simulink model "MODEL_nieliniowy_prevprevprev"  (R2020b)
settings: Solver=VariableStepAuto  StartTime=0.0  StopTime=1200  RelTol=1e-3
values from neighbouring files (symbols this model uses):
  c1 = 1    [zadanie_inaczej.m]
  c2 = 2    [zadanie_inaczej.m]
  K = 0.02    [zadanie_inaczej.m]
  S = 1    [zadanie_inaczej.m]
settings Model: PauseTimes=0  Creator=Adam  LastModifiedBy=Adam

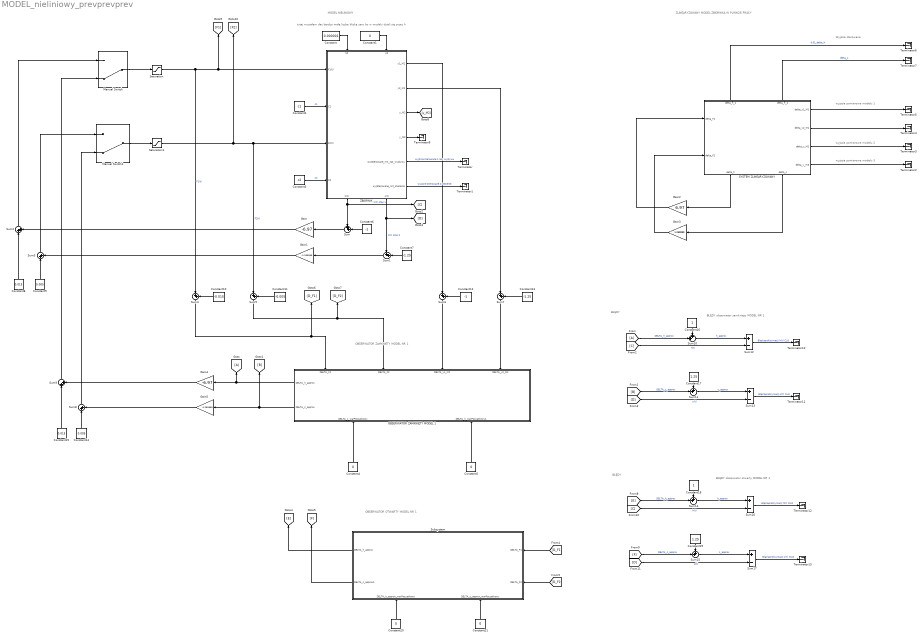
== system MODEL_nieliniowy_prevprevprev ==
  note: BŁĘDY obserwator zamknięty MODEL NR 1
  note: OBSERWATOR ZAMKNIETY MODEL NR 1
  note: BŁĘDY
  note: tutaj musiałem dać bardzo małą liczbe bliską zero bo w modelu dzieli się przez h
  note: wyjscia pomiarowe modelu 3
  note: ZLINEARYZOWANY MODEL ZBIORNIKA W PUNKCIE PRACY
  note: wyjscia pomiarowe modelu 1
  note: wyjscia pomiarowe modelu 2
  note: Wyjścia sterowane
  note: MODEL NIELINIOWY
  note: BŁĘDY
  note: BŁĘDY obserwator otwarty
      | MODEL NR 1
  note: OBSERWATOR OTWARTY MODEL NR 1
  Constant : Constant  Value=0.000001
  Constant{1,4..5,20..21} (5 alike) : Constant  Value=0
  Constant10 : Constant  Value=-0.015
  Constant11 : Constant  Value=-0.005
  Constant12 : Constant  Value=-1
  Constant13 : Constant  Value=-1.25
  Constant14 : Constant  Value=0.005
  Constant15 : Constant  Value=0.015
  Constant16 : Constant
  Constant17 : Constant  Value=1.25
  Constant18 : Constant
  Constant19 : Constant  Value=1.25
  Constant2 : Constant  Value=c1
  Constant3 : Constant  Value=c2
  Constant6 : Constant  Value=-1
  Constant7 : Constant  Value=-1.25
  Constant8 : Constant  Value=0.015
  Constant9 : Constant  Value=0.005
  Gain : Gain  Gain=-6.97
  Gain1 : Gain  Gain=-1.269999
  Gain2 : Gain  Gain=6.97
  Gain3 : Gain  Gain=1.269999
  Gain4 : Gain  Gain=-6.97
  Gain5 : Gain  Gain=-1.269999
  Manual Switch : ManualSwitch  CurrentSetting=0
  Manual Switch1 : ManualSwitch  CurrentSetting=0
  OBSERWATOR ZAMKNIĘTY MODEL 1 : Subsystem
      settings: PortSchema="{\"entries\":[{\"content\":{\"sides\":[{\"content\":{\"connectorIds\":[]},\"type\":\"ConnectorPlacement.EquallySpacedRectSide\",\"uuid\":\"df9a0dc1-4b9c-40dc-a757-6b1a6b9aa6ed\"},{\"content\":{\"connectorIds\":[\"Out1\",\"Out2\"],\"side\":\"RIGHT\"},\"type\":\"ConnectorPlacement.EquallySpacedRectSide\",\"uuid\":\"5cba16cf-a15e-4045-92be-3e6ecad2ae7f\"},{\"content\":{\"connectorIds\":[\"In1\",\"In2\",\"In3\",\"In4\"],\"side\":\"TOP\"},\"type\":\"ConnectorPlacement.EquallySpacedRectSide\",\"uuid\":\"e348609f-8070-4092-8204-65a83adf26dd\"},{\"content\":{\"connectorIds\":[\"In5\",\"In6\"],\"side\":\"BOTTOM\"},\"type\":\"ConnectorPlacement.EquallySpacedRectSide\",\"uuid\":\"61fc9fd5-86f3-4303-bf38-07e595d55bb3\"},{\"content\":{\"connectorIds\":[],\"side\":\"HIDDEN\"},\"type\":\"ConnectorPlacement.EquallySpacedRectSide\",\"uuid\":\"65a64511-4a73-4e57-a778-b63fa28d7d79\"}]},\"type\":\"ConnectorPlacement.EquallySpacedConnector\",\"uuid\":\"74f27241-a0e0-45b7-b881-233bfa2226d6\"}],\"packageUris\":[\"http://schema.mathworks.com/mf0/Connector/R2020b\"],\"version\":\"1.0\"}"
  SYSTEM ZLINEARYZOWANY : Subsystem
      settings: PortSchema="{\"entries\":[{\"content\":{\"sides\":[{\"content\":{\"connectorIds\":[\"In1\",\"In2\"]},\"type\":\"ConnectorPlacement.EquallySpacedRectSide\",\"uuid\":\"d54e25d2-cd73-45e0-9808-ca3ea5dc6cf7\"},{\"content\":{\"connectorIds\":[\"Out1\",\"Out2\",\"Out3\",\"Out4\"],\"side\":\"RIGHT\"},\"type\":\"ConnectorPlacement.EquallySpacedRectSide\",\"uuid\":\"8f74ab67-fea9-4695-8f57-14f1d1e6aeae\"},{\"content\":{\"connectorIds\":[\"Out7\",\"Out8\"],\"side\":\"TOP\"},\"type\":\"ConnectorPlacement.EquallySpacedRectSide\",\"uuid\":\"7e2d5216-70d7-4fc4-9048-f9922785c559\"},{\"content\":{\"connectorIds\":[\"Out5\",\"Out6\"],\"side\":\"BOTTOM\"},\"type\":\"ConnectorPlacement.EquallySpacedRectSide\",\"uuid\":\"2e3112e0-8f75-4fde-8abe-6ce63d8f82f0\"},{\"content\":{\"connectorIds\":[],\"side\":\"HIDDEN\"},\"type\":\"ConnectorPlacement.EquallySpacedRectSide\",\"uuid\":\"0c231cea-7ad8-44fc-a940-5c2cadec50e3\"}]},\"type\":\"ConnectorPlacement.EquallySpacedConnector\",\"uuid\":\"51c5d8a6-0e0c-4ace-bfb7-5845e71f886b\"}],\"packageUris\":[\"http://schema.mathworks.com/mf0/Connector/R2020b\"],\"version\":\"1.0\"}"
  Saturation : Saturate  UpperLimit=inf  LowerLimit=0
  Saturation1 : Saturate  UpperLimit=inf  LowerLimit=0
  Subsystem : Subsystem
      settings: PortSchema="{\"entries\":[{\"content\":{\"sides\":[{\"content\":{\"connectorIds\":[\"In1\",\"In2\"]},\"type\":\"ConnectorPlacement.EquallySpacedRectSide\",\"uuid\":\"9da57aff-d8ed-41ac-be0f-7bb7d22a2d6d\"},{\"content\":{\"connectorIds\":[\"Out1\",\"Out2\"],\"side\":\"RIGHT\"},\"type\":\"ConnectorPlacement.EquallySpacedRectSide\",\"uuid\":\"4a485f9a-c196-4acf-9f6f-00c6dbb16d48\"},{\"content\":{\"connectorIds\":[],\"side\":\"TOP\"},\"type\":\"ConnectorPlacement.EquallySpacedRectSide\",\"uuid\":\"007a8443-3490-401f-88cc-683f6a14c27c\"},{\"content\":{\"connectorIds\":[\"In3\",\"In4\"],\"side\":\"BOTTOM\"},\"type\":\"ConnectorPlacement.EquallySpacedRectSide\",\"uuid\":\"09129c57-b904-461c-b339-9340df3751d4\"},{\"content\":{\"connectorIds\":[],\"side\":\"HIDDEN\"},\"type\":\"ConnectorPlacement.EquallySpacedRectSide\",\"uuid\":\"f4f5cd58-23cc-4937-8552-2264c9543629\"}]},\"type\":\"ConnectorPlacement.EquallySpacedConnector\",\"uuid\":\"c4e5adba-5bf6-49ba-a33f-504984928f5e\"}],\"packageUris\":[\"http://schema.mathworks.com/mf0/Connector/R2020b\"],\"version\":\"1.0\"}"
  Sum{,1,10..11,14..15} (6 alike) : Sum  Inputs=++|
  Sum{12..13,16..17} (4 alike) : Sum  Inputs=+-
  Sum{2..9} (8 alike) : Sum  Inputs=|++
  Terminator{,1..7,9..13} (13 alike) : Terminator
  ZBIORNIK : Subsystem
      settings: PortSchema="{\"entries\":[{\"content\":{\"sides\":[{\"content\":{\"connectorIds\":[\"In1\",\"In2\",\"In3\",\"In4\"]},\"type\":\"ConnectorPlacement.EquallySpacedRectSide\",\"uuid\":\"d7534cdc-3a83-4663-9669-478cefb7ba54\"},{\"content\":{\"connectorIds\":[\"Out1\",\"Out2\",\"Out3\",\"Out4\",\"Out5\",\"Out6\"],\"side\":\"RIGHT\"},\"type\":\"ConnectorPlacement.EquallySpacedRectSide\",\"uuid\":\"43aa4112-be2a-4a64-a360-86159253405e\"},{\"content\":{\"connectorIds\":[\"In5\",\"In6\"],\"side\":\"TOP\"},\"type\":\"ConnectorPlacement.EquallySpacedRectSide\",\"uuid\":\"a87f647c-d073-49ff-8fa7-c7401791c269\"},{\"content\":{\"connectorIds\":[\"Out7\",\"Out8\"],\"side\":\"BOTTOM\"},\"type\":\"ConnectorPlacement.EquallySpacedRectSide\",\"uuid\":\"6d6aa66b-079d-45b1-a0b1-1cea6131b53f\"},{\"content\":{\"connectorIds\":[],\"side\":\"HIDDEN\"},\"type\":\"ConnectorPlacement.EquallySpacedRectSide\",\"uuid\":\"1d6cc66c-e8b9-4690-8052-ee4d3cbcc1b2\"}]},\"type\":\"ConnectorPlacement.EquallySpacedConnector\",\"uuid\":\"a7312018-d894-48d8-963b-edf04426afa5\"}],\"packageUris\":[\"http://schema.mathworks.com/mf0/Connector/R2020b\"],\"version\":\"1.0\"}"
  wires:
  Constant2/1 -> ZBIORNIK/2(C1)  "c1"
  Constant3/1 -> ZBIORNIK/4(C2)  "c2"
  Constant1/1 -> ZBIORNIK/6(c0)
  Constant/1 -> ZBIORNIK/5(h0)
  SYSTEM ZLINEARYZOWANY/7(delta_fi_1) -> Terminator6/1  "0.01_delta_h"
  SYSTEM ZLINEARYZOWANY/1(delta_y1_M1) -> Terminator5/1
  SYSTEM ZLINEARYZOWANY/2(delta_y2_M1) -> Terminator4/1
  SYSTEM ZLINEARYZOWANY/3(delta_y_M2) -> Terminator3/1
  SYSTEM ZLINEARYZOWANY/4(delta_y_m3) -> Terminator2/1
  SYSTEM ZLINEARYZOWANY/8(delta_fi_2) -> Terminator7/1  "delta_c"
  ZBIORNIK/7(h(t)) -> [C], Sum/1  "h(t) stan 1"
  Sum/1 -> Gain/1
  Constant6/1 -> Sum/2
  Constant7/1 -> Sum1/2
  ZBIORNIK/8(c(t)) -> Sum1/1, [D]  "c(t) stan 2"
  Sum1/1 -> Gain1/1
  Gain/1 -> Sum2/2
  Gain1/1 -> Sum3/2
  Constant8/1 -> Sum2/1
  Constant9/1 -> Sum3/1
  ZBIORNIK/5(wyjSterowane_nr1_nat_wyplywu) -> Terminator/1  "wyjście sterowane 1 nat. wyplywu"
  ZBIORNIK/6(wyjSterowane_nr2_stezenie) -> Terminator1/1  "wyjście sterowane 2 stezenie"
  SYSTEM ZLINEARYZOWANY/5(delta_h) -> Gain2/1
  SYSTEM ZLINEARYZOWANY/6(delta_c) -> Gain3/1
  Gain2/1 -> SYSTEM ZLINEARYZOWANY/1(delta_F1)
  Gain3/1 -> SYSTEM ZLINEARYZOWANY/2(delta_F2)
  Saturation/1 -> [F1], ZBIORNIK/1(F1(t)), Sum4/1  "F1(t)"
  Manual Switch/1 -> Saturation/1
  Manual Switch1/1 -> Saturation1/1
  Saturation1/1 -> Sum5/1, ZBIORNIK/3(F2(t)), [F2]  "F2(t)"
  Constant10/1 -> Sum4/2
  Constant11/1 -> Sum5/2
  Sum4/1 -> [D_F1], OBSERWATOR ZAMKNIĘTY MODEL 1/4(DELTA_F1)
  Sum5/1 -> OBSERWATOR ZAMKNIĘTY MODEL 1/3(DELTA_F2), [D_F2]
  Constant12/1 -> Sum6/2
  Constant13/1 -> Sum7/2
  ZBIORNIK/1(y1_M1) -> Sum6/1
  ZBIORNIK/2(y2_M1) -> Sum7/1
  Sum6/1 -> OBSERWATOR ZAMKNIĘTY MODEL 1/2(DELTA_y1_M1)
  Sum7/1 -> OBSERWATOR ZAMKNIĘTY MODEL 1/1(DELTA_y2_M2)
  OBSERWATOR ZAMKNIĘTY MODEL 1/2(DELTA_c_approx) -> [B], Gain5/1
  OBSERWATOR ZAMKNIĘTY MODEL 1/1(DELTA_h_approx) -> [A], Gain4/1
  Constant14/1 -> Sum8/1
  Gain5/1 -> Sum8/2
  Constant15/1 -> Sum9/1
  Gain4/1 -> Sum9/2
  Sum2/1 -> Manual Switch/1
  Sum3/1 -> Manual Switch1/1
  Sum9/1 -> Manual Switch/2
  Sum8/1 -> Manual Switch1/2
  Constant4/1 -> OBSERWATOR ZAMKNIĘTY MODEL 1/6(DELTA_c_warPoczatkowy)
  Constant5/1 -> OBSERWATOR ZAMKNIĘTY MODEL 1/5(DELTA_h_warPoczatkowy1)
  ZBIORNIK/3(y_M2) -> [y_M2]
  ZBIORNIK/4(y_M3) -> Terminator9/1
  [A] -> Sum10/2  "DELTA_h_approx"
  [B] -> Sum11/2  "DELTA_c_approx"
  [C] -> Sum12/2  "h(t)"
  [D] -> Sum13/2  "c(t)"
  Constant16/1 -> Sum10/1
  Constant17/1 -> Sum11/1
  Sum10/1 -> Sum12/1  "h_approx"
  Sum11/1 -> Sum13/1  "c_approx"
  Sum13/1 -> Terminator11/1  "Błąd aproksymacji c(t) CLO"
  Sum12/1 -> Terminator10/1  "Błąd aproksymacji h(t) CLO"
  Subsystem/1(DELTA_h_approx) -> [E]
  Subsystem/2(DELTA_c_approx1) -> [F]
  [D_F1] -> Subsystem/1(DELTA_F1)
  [D_F2] -> Subsystem/2(DELTA_F2)
  Sum16/1 -> Terminator12/1  "Błąd aproksymacji h(t) OLO"
  Sum14/1 -> Sum16/1  "h_approx"
  Constant18/1 -> Sum14/1
  Sum15/1 -> Sum17/1  "c_approx"
  Constant19/1 -> Sum15/1
  [D] -> Sum17/2  "c(t)"
  Sum17/1 -> Terminator13/1  "Błąd aproksymacji c(t) OLO"
  [C] -> Sum16/2  "h(t)"
  [E] -> Sum14/2  "DELTA_h_approx"
  [F] -> Sum15/2  "DELTA_c_approx"
  Constant20/1 -> Subsystem/4(DELTA_h_approx_warPoczatkowy)
  Constant21/1 -> Subsystem/3(DELTA_c_approx_warPoczatkowy)

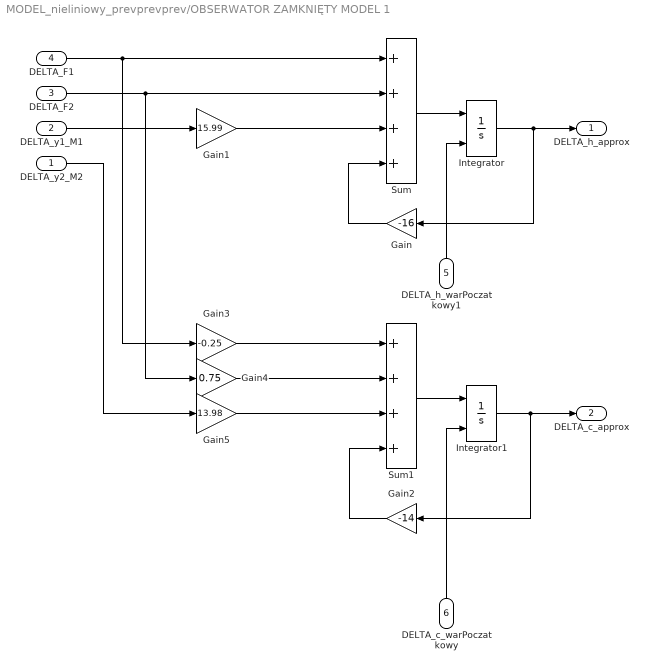
== system MODEL_nieliniowy_prevprevprev/OBSERWATOR ZAMKNIĘTY MODEL 1 ==
  DELTA_y2_M2 : Inport
  DELTA_y1_M1 : Inport  Port=2
  DELTA_F2 : Inport  Port=3
  DELTA_F1 : Inport  Port=4
  DELTA_h_warPoczatkowy1 : Inport  Port=5
  DELTA_c_warPoczatkowy : Inport  Port=6
  Gain : Gain  Gain=-16
  Gain1 : Gain  Gain=15.99
  Gain2 : Gain  Gain=-14
  Gain3 : Gain  Gain=-0.25
  Gain4 : Gain  Gain=0.75
  Gain5 : Gain  Gain=13.98
  Integrator : Integrator  InitialConditionSource=external
  Integrator1 : Integrator  InitialConditionSource=external
  Sum : Sum  Inputs=++++
  Sum1 : Sum  Inputs=++++
  DELTA_h_approx : Outport
  DELTA_c_approx : Outport  Port=2
  wires:
  Integrator/1 -> DELTA_h_approx/1, Gain/1
  Sum/1 -> Integrator/1
  Gain/1 -> Sum/4
  DELTA_F1/1 -> Gain3/1, Sum/1
  DELTA_F2/1 -> Sum/2, Gain4/1
  DELTA_y1_M1/1 -> Gain1/1
  Gain1/1 -> Sum/3
  Integrator1/1 -> DELTA_c_approx/1, Gain2/1
  Sum1/1 -> Integrator1/1
  Gain2/1 -> Sum1/4
  Gain3/1 -> Sum1/1
  Gain4/1 -> Sum1/2
  DELTA_y2_M2/1 -> Gain5/1
  Gain5/1 -> Sum1/3
  DELTA_c_warPoczatkowy/1 -> Integrator1/2
  DELTA_h_warPoczatkowy1/1 -> Integrator/2

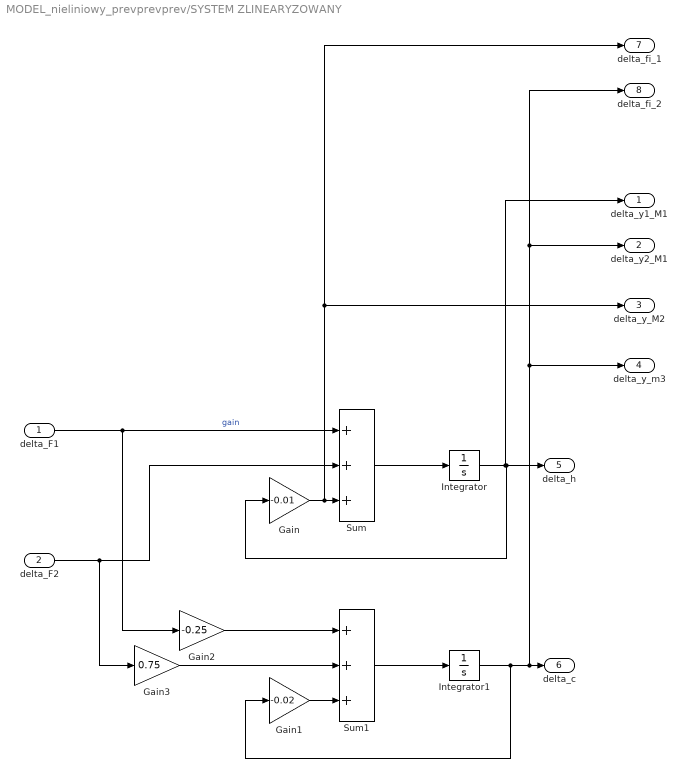
== system MODEL_nieliniowy_prevprevprev/SYSTEM ZLINEARYZOWANY ==
  delta_F1 : Inport
  delta_F2 : Inport  Port=2
  Gain : Gain  Gain=-0.01
  Gain1 : Gain  Gain=-0.02
  Gain2 : Gain  Gain=-0.25
  Gain3 : Gain  Gain=0.75
  Integrator : Integrator
  Integrator1 : Integrator
  Sum : Sum  Inputs=+++
  Sum1 : Sum  Inputs=+++
  delta_y1_M1 : Outport
  delta_y2_M1 : Outport  Port=2
  delta_y_M2 : Outport  Port=3
  delta_y_m3 : Outport  Port=4
  delta_h : Outport  Port=5
  delta_c : Outport  Port=6
  delta_fi_1 : Outport  Port=7
  delta_fi_2 : Outport  Port=8
  wires:
  Integrator1/1 -> delta_y_m3/1, delta_y2_M1/1, delta_fi_2/1, delta_c/1, Gain1/1
  Integrator/1 -> delta_y1_M1/1, Gain/1, delta_h/1
  Gain/1 -> delta_y_M2/1, delta_fi_1/1, Sum/3
  Sum/1 -> Integrator/1
  delta_F1/1 -> Gain2/1, Sum/1  "gain"
  delta_F2/1 -> Gain3/1, Sum/2
  Sum1/1 -> Integrator1/1
  Gain1/1 -> Sum1/3
  Gain2/1 -> Sum1/1
  Gain3/1 -> Sum1/2

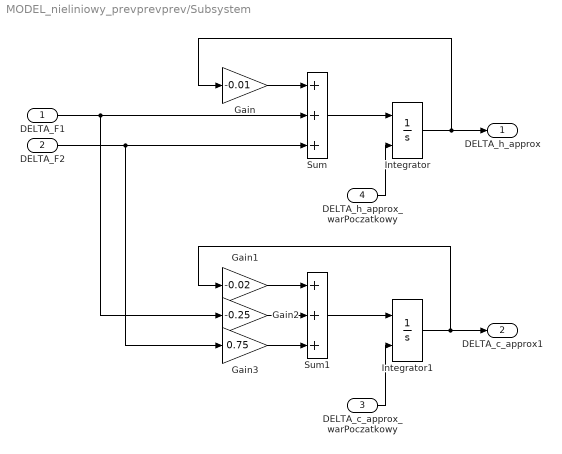
== system MODEL_nieliniowy_prevprevprev/Subsystem ==
  DELTA_F1 : Inport
  DELTA_F2 : Inport  Port=2
  DELTA_c_approx_warPoczatkowy : Inport  Port=3
  DELTA_h_approx_warPoczatkowy : Inport  Port=4
  Gain : Gain  Gain=-0.01
  Gain1 : Gain  Gain=-0.02
  Gain2 : Gain  Gain=-0.25
  Gain3 : Gain  Gain=0.75
  Integrator : Integrator  InitialConditionSource=external
  Integrator1 : Integrator  InitialConditionSource=external
  Sum : Sum  Inputs=+++
  Sum1 : Sum  Inputs=+++
  DELTA_h_approx : Outport
  DELTA_c_approx1 : Outport  Port=2
  wires:
  Gain/1 -> Sum/1
  Sum/1 -> Integrator/1
  Integrator/1 -> Gain/1, DELTA_h_approx/1
  DELTA_F1/1 -> Gain2/1, Sum/2
  DELTA_F2/1 -> Gain3/1, Sum/3
  Sum1/1 -> Integrator1/1
  Integrator1/1 -> Gain1/1, DELTA_c_approx1/1
  Gain1/1 -> Sum1/1
  Gain2/1 -> Sum1/2
  Gain3/1 -> Sum1/3
  DELTA_h_approx_warPoczatkowy/1 -> Integrator/2
  DELTA_c_approx_warPoczatkowy/1 -> Integrator1/2

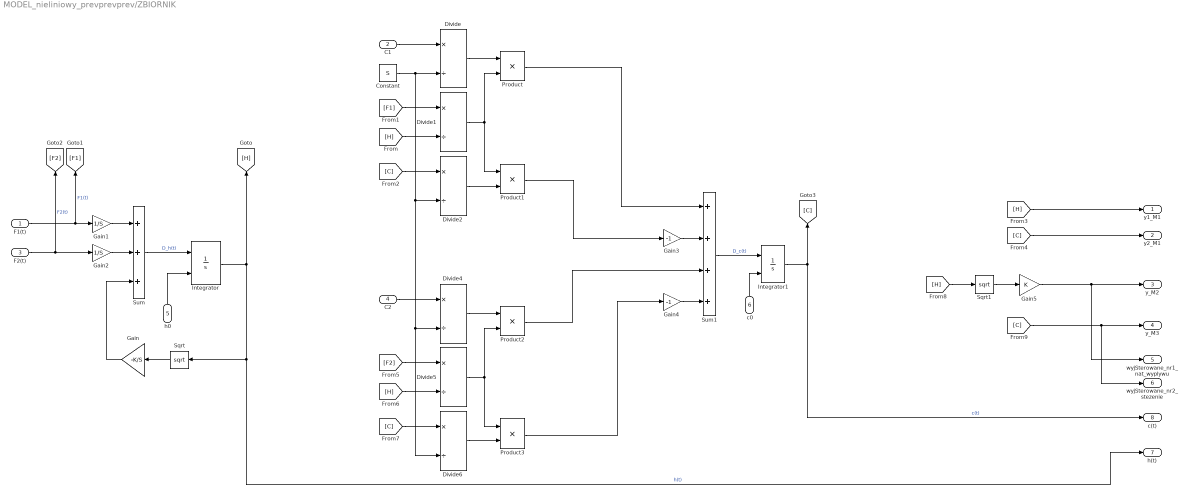
== system MODEL_nieliniowy_prevprevprev/ZBIORNIK ==
  F1(t) : Inport
  C1 : Inport  Port=2
  F2(t) : Inport  Port=3
  C2 : Inport  Port=4
  h0 : Inport  Port=5
  c0 : Inport  Port=6
  Constant : Constant  Value=S
  Divide{,1..2,4..6} (6 alike) : Product  Inputs=*/
  Gain : Gain  Gain=-K/S
  Gain1 : Gain  Gain=1/S
  Gain2 : Gain  Gain=1/S
  Gain3 : Gain  Gain=-1
  Gain4 : Gain  Gain=-1
  Gain5 : Gain  Gain=K
  Integrator : Integrator  InitialConditionSource=external
  Integrator1 : Integrator  InitialConditionSource=external
  Product{,1..3} (4 alike) : Product
  Sqrt : Sqrt  OutputSignalType=real  SaturateOnIntegerOverflow=on
  Sqrt1 : Sqrt  SaturateOnIntegerOverflow=on
  Sum : Sum  Inputs=+++
  Sum1 : Sum  Inputs=++++
  y1_M1 : Outport
  y2_M1 : Outport  Port=2
  y_M2 : Outport  Port=3
  y_M3 : Outport  Port=4
  wyjSterowane_nr1_nat_wyplywu : Outport  Port=5
  wyjSterowane_nr2_stezenie : Outport  Port=6
  h(t) : Outport  Port=7
  c(t) : Outport  Port=8
  wires:
  C2/1 -> Divide4/1
  Product1/1 -> Gain3/1
  Product2/1 -> Sum1/3
  Divide5/1 -> Product3/1, Product2/2
  Gain4/1 -> Sum1/4
  [F2] -> Divide5/1
  Constant/1 -> Divide2/2, Divide4/2, Divide6/2, Divide/2
  C1/1 -> Divide/1
  Sum1/1 -> Integrator1/1  "D_c(t)"
  Product3/1 -> Gain4/1
  F1(t)/1 -> Gain1/1, [F1]  "F1(t)"
  [H] -> Divide1/2
  Gain1/1 -> Sum/1
  F2(t)/1 -> Gain2/1, [F2]  "F2(t)"
  Gain3/1 -> Sum1/2
  [C] -> Divide6/1
  Sum/1 -> Integrator/1  "D_h(t)"
  Divide4/1 -> Product2/1
  Sqrt/1 -> Gain/1
  Integrator1/1 -> [C], c(t)/1  "c(t)"
  Gain2/1 -> Sum/2
  Divide1/1 -> Product1/1, Product/2
  [C] -> Divide2/1
  [F1] -> Divide1/1
  [H] -> Divide5/2
  Divide6/1 -> Product3/2
  Divide/1 -> Product/1
  Product/1 -> Sum1/1
  h0/1 -> Integrator/2
  c0/1 -> Integrator1/2
  Divide2/1 -> Product1/2
  Integrator/1 -> Sqrt/1, h(t)/1, [H]  "h(t)"
  Gain/1 -> Sum/3
  [H] -> y1_M1/1
  [C] -> y2_M1/1
  Sqrt1/1 -> Gain5/1
  Gain5/1 -> wyjSterowane_nr1_nat_wyplywu/1, y_M2/1
  [H] -> Sqrt1/1
  [C] -> y_M3/1, wyjSterowane_nr2_stezenie/1
